simulink model "DT_GeneralFSM"  (R2025b)
settings: Solver=VariableStepAuto  StartTime=0.0  StopTime=1343.25  RelTol=1e-3
values from neighbouring files (symbols this model uses):
  feeddata = struct()    [DT_generatedata.m]    (also in DT_readdata.m)
  GSmode = input(['Choose the model type\n'                  '   [1] Kinetic + Genome-Scale Model\n'                  '   [2] Kinetic Only\n'                  'Response: '])    [DT_Run_GSA.m]    (also in DT_run.m; DT_run_OptimizeCOGs.m = 0; DT_run_ParaEst.m)
undefined symbols (not defined in the file or in its folder): V1, V2, V3, V4, V5, V6, V7
libraries: DT_Library x30
settings Model: DataDictionary=DT_types.sldd  SimulationMode=accelerator  PacingRate=0.100000  Creator=fenix  LastModifiedBy=Fenix
settings DebuggingCC: AlgebraicLoopMsg=error  UnitsInconsistencyMsg=none

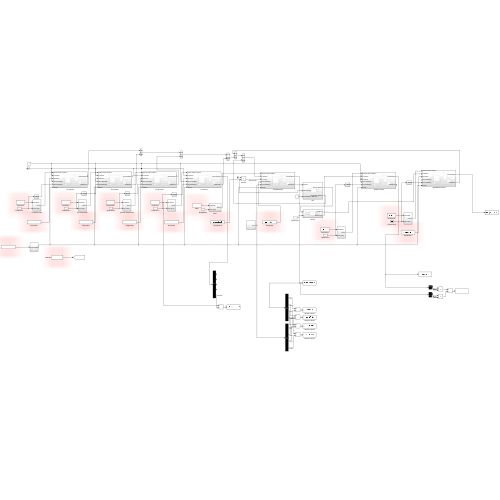
[thumbnail: Simulink's stored preview of the top-level diagram]
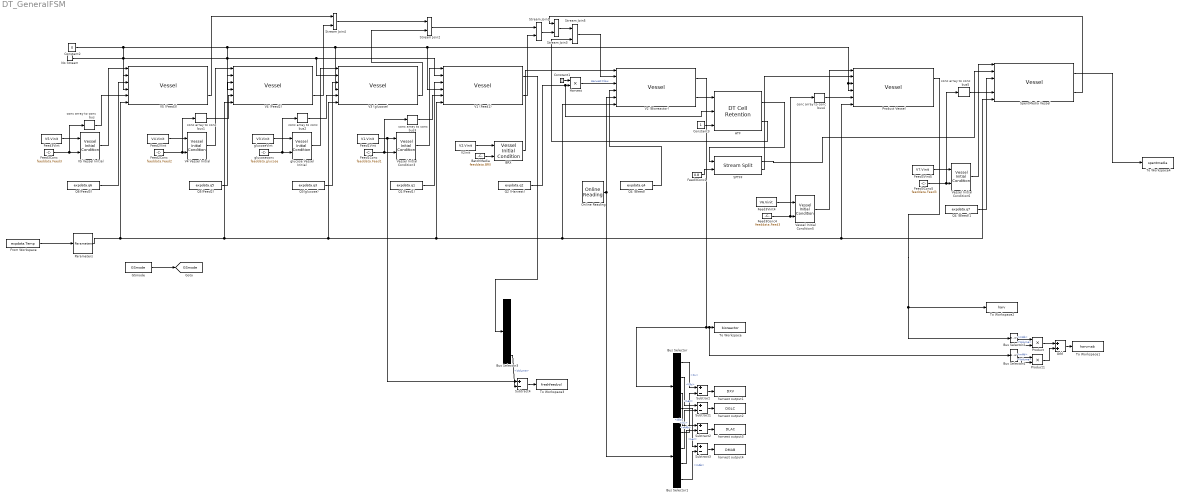
== system DT_GeneralFSM ==
  ATF : DT_Library/DT Cell Retention  SystemSampleTime=-1  VariantActivationTime=update diagram  EmptyChoice=off  PassThrough=off  PassThroughVariantControl=(default)  EmptyChoiceVariantControl=(default)  AllowFlexibleInterface=on  Latency=0  AutoFrameSizeCalculation=off
  Add : Sum
  BRX : DT_Library/Vessel Initial Condition  SystemSampleTime=-1  VariantActivationTime=update diagram  EmptyChoice=off  PassThrough=off  PassThroughVariantControl=(default)  EmptyChoiceVariantControl=(default)  AllowFlexibleInterface=on  Latency=0  AutoFrameSizeCalculation=off
  BatchMedia : Constant  Value=feeddata.BRX
  Bus Selector : BusSelector  OutputSignals=conc.Xv,conc.Glc,conc.Lac,conc.mAb
  Bus Selector1 : BusSelector  OutputSignals=Xv,Glc,Lac,mAb
  Bus Selector2 : BusSelector  OutputSignals=conc.Xv,conc.Glc,conc.Lac,conc.mAb,Volume
  Bus Selector3 : BusSelector  OutputSignals=conc.Xv,conc.Glc,conc.Lac,conc.mAb,Volume
  Bus Selector4 : BusSelector  OutputSignals=conc.Xv,conc.Glc,conc.Lac,conc.mAb,Volume
  Constant1 : Constant  Value=2
  Constant2 : Constant  Value=0
  Constant3 : Constant
  Feed1Conc : Constant  Value=feeddata.Feed1
  Feed1Vint : Constant  Value=V1.Vinit
  Feed2Conc : Constant  Value=feeddata.Feed2
  Feed2Vint : Constant  Value=V4.Vinit
  Feed3Conc : Constant  Value=feeddata.Feed3
  Feed3Conc1 : Constant  Value=0.8
  Feed3Conc4 : Constant  Value=feeddata.Feed3
  Feed3Conc5 : Constant  Value=feeddata.Feed3
  Feed3Vint : Constant  Value=V5.Vinit
  Feed3Vint4 : Constant  Value=V6.Vinit
  Feed3Vint5 : Constant  Value=V7.Vinit
  From Workspace : FromWorkspace  VariableName=expdata.Temp  Interpolate=off  OutputAfterFinalValue=Holding final value
  GSmode : Constant  Value=GSmode
  Harvest : Product
  No Stream : DT_Library/No Stream  SystemSampleTime=-1  VariantActivationTime=update diagram  EmptyChoice=off  PassThrough=off  PassThroughVariantControl=(default)  EmptyChoiceVariantControl=(default)  AllowFlexibleInterface=on  Latency=0  AutoFrameSizeCalculation=off
  Online Reading : DT_Library/Online Reading  SystemSampleTime=-1  VariantActivationTime=update diagram  EmptyChoice=off  PassThrough=off  PassThroughVariantControl=(default)  EmptyChoiceVariantControl=(default)  AllowFlexibleInterface=on  Latency=0  AutoFrameSizeCalculation=off
  Parameters : DT_Library/Parameters  SystemSampleTime=-1  VariantActivationTime=update diagram  EmptyChoice=off  PassThrough=off  PassThroughVariantControl=(default)  EmptyChoiceVariantControl=(default)  AllowFlexibleInterface=on  Latency=0  AutoFrameSizeCalculation=off
  Product : Product
  Product Vessel : DT_Library/Vessel  SystemSampleTime=-1  VariantActivationTime=update diagram  EmptyChoice=off  PassThrough=off  PassThroughVariantControl=(default)  EmptyChoiceVariantControl=(default)  AllowFlexibleInterface=on  Latency=0  AutoFrameSizeCalculation=off
  Product1 : Product
  Q1(Feed1) : FromWorkspace  VariableName=expdata.q1  Interpolate=off  OutputAfterFinalValue=Holding final value
  Q2 (Harvest) : FromWorkspace  VariableName=expdata.q2  Interpolate=off  OutputAfterFinalValue=Holding final value
  Q3(glucose) : FromWorkspace  VariableName=expdata.q3  Interpolate=off  OutputAfterFinalValue=Holding final value
  Q4 (Bleed) : FromWorkspace  VariableName=expdata.q4  Interpolate=off  OutputAfterFinalValue=Holding final value
  Q4 (Bleed)1 : FromWorkspace  VariableName=expdata.q7  Interpolate=off  OutputAfterFinalValue=Holding final value
  Q5(Feed2) : FromWorkspace  VariableName=expdata.q5  Interpolate=off  OutputAfterFinalValue=Holding final value
  Q6(Feed3) : FromWorkspace  VariableName=expdata.q6  Interpolate=off  OutputAfterFinalValue=Holding final value
  SPTFF : DT_Library/Stream Split  SystemSampleTime=-1  VariantActivationTime=update diagram  EmptyChoice=off  PassThrough=off  PassThroughVariantControl=(default)  EmptyChoiceVariantControl=(default)  AllowFlexibleInterface=on  Latency=0  AutoFrameSizeCalculation=off
  SpentMedia Vessel : DT_Library/Vessel  SystemSampleTime=-1  VariantActivationTime=update diagram  EmptyChoice=off  PassThrough=off  PassThroughVariantControl=(default)  EmptyChoiceVariantControl=(default)  AllowFlexibleInterface=on  Latency=0  AutoFrameSizeCalculation=off
  Stream Join{1..5} (5 alike) : DT_Library/Stream Join  SystemSampleTime=-1  VariantActivationTime=update diagram  EmptyChoice=off  PassThrough=off  PassThroughVariantControl=(default)  EmptyChoiceVariantControl=(default)  AllowFlexibleInterface=on  Latency=0  AutoFrameSizeCalculation=off
  Subtract{,1..4} (5 alike) : Sum  Inputs=+-
  To Workspace : ToWorkspace  VariableName=bioreactor  SaveFormat=Timeseries  SampleTime=-1
  To Workspace1 : ToWorkspace  VariableName=harvmab  SaveFormat=Timeseries  SampleTime=-1
  To Workspace2 : ToWorkspace  VariableName=harv  SaveFormat=Timeseries  SampleTime=-1
  To Workspace3 : ToWorkspace  VariableName=freshfeedvol  SaveFormat=Timeseries  SampleTime=-1
  To Workspace4 : ToWorkspace  VariableName=spentmedia  SaveFormat=Timeseries  SampleTime=-1
  V1 (Feed1) : DT_Library/Vessel  SystemSampleTime=-1  VariantActivationTime=update diagram  EmptyChoice=off  PassThrough=off  PassThroughVariantControl=(default)  EmptyChoiceVariantControl=(default)  AllowFlexibleInterface=on  Latency=0  AutoFrameSizeCalculation=off
  V2 (Bioreactor) : DT_Library/Vessel  SystemSampleTime=-1  VariantActivationTime=update diagram  EmptyChoice=off  PassThrough=off  PassThroughVariantControl=(default)  EmptyChoiceVariantControl=(default)  AllowFlexibleInterface=on  Latency=0  AutoFrameSizeCalculation=off
  V2init : Constant  Value=V2.Vinit
  V3 (glucose) : DT_Library/Vessel  SystemSampleTime=-1  VariantActivationTime=update diagram  EmptyChoice=off  PassThrough=off  PassThroughVariantControl=(default)  EmptyChoiceVariantControl=(default)  AllowFlexibleInterface=on  Latency=0  AutoFrameSizeCalculation=off
  V4 (Feed2) : DT_Library/Vessel  SystemSampleTime=-1  VariantActivationTime=update diagram  EmptyChoice=off  PassThrough=off  PassThroughVariantControl=(default)  EmptyChoiceVariantControl=(default)  AllowFlexibleInterface=on  Latency=0  AutoFrameSizeCalculation=off
  V4 Vessel Initial : DT_Library/Vessel Initial Condition  SystemSampleTime=-1  VariantActivationTime=update diagram  EmptyChoice=off  PassThrough=off  PassThroughVariantControl=(default)  EmptyChoiceVariantControl=(default)  AllowFlexibleInterface=on  Latency=0  AutoFrameSizeCalculation=off
  V5 (Feed3) : DT_Library/Vessel  SystemSampleTime=-1  VariantActivationTime=update diagram  EmptyChoice=off  PassThrough=off  PassThroughVariantControl=(default)  EmptyChoiceVariantControl=(default)  AllowFlexibleInterface=on  Latency=0  AutoFrameSizeCalculation=off
  "V5 Vessel Initial " : DT_Library/Vessel Initial Condition  SystemSampleTime=-1  VariantActivationTime=update diagram  EmptyChoice=off  PassThrough=off  PassThroughVariantControl=(default)  EmptyChoiceVariantControl=(default)  AllowFlexibleInterface=on  Latency=0  AutoFrameSizeCalculation=off
  Vessel Initial Condition3 : DT_Library/Vessel Initial Condition  SystemSampleTime=-1  VariantActivationTime=update diagram  EmptyChoice=off  PassThrough=off  PassThroughVariantControl=(default)  EmptyChoiceVariantControl=(default)  AllowFlexibleInterface=on  Latency=0  AutoFrameSizeCalculation=off
  Vessel Initial Condition5 : DT_Library/Vessel Initial Condition  SystemSampleTime=-1  VariantActivationTime=update diagram  EmptyChoice=off  PassThrough=off  PassThroughVariantControl=(default)  EmptyChoiceVariantControl=(default)  AllowFlexibleInterface=on  Latency=0  AutoFrameSizeCalculation=off
  Vessel Initial Condition6 : DT_Library/Vessel Initial Condition  SystemSampleTime=-1  VariantActivationTime=update diagram  EmptyChoice=off  PassThrough=off  PassThroughVariantControl=(default)  EmptyChoiceVariantControl=(default)  AllowFlexibleInterface=on  Latency=0  AutoFrameSizeCalculation=off
  conc array to conc bus{,1..5} (6 alike) : DT_Library/conc array to conc bus  SystemSampleTime=-1  VariantActivationTime=update diagram  EmptyChoice=off  PassThrough=off  PassThroughVariantControl=(default)  EmptyChoiceVariantControl=(default)  AllowFlexibleInterface=on  Latency=0  AutoFrameSizeCalculation=off
  glucose Vessel Initial : DT_Library/Vessel Initial Condition  SystemSampleTime=-1  VariantActivationTime=update diagram  EmptyChoice=off  PassThrough=off  PassThroughVariantControl=(default)  EmptyChoiceVariantControl=(default)  AllowFlexibleInterface=on  Latency=0  AutoFrameSizeCalculation=off
  glucoseVint : Constant  Value=V3.Vinit
  glucoseconc : Constant  Value=feeddata.glucose
  harvest output1 : ToWorkspace  VariableName=DXV  SaveFormat=Timeseries  SampleTime=-1
  harvest output2 : ToWorkspace  VariableName=DGLC  SaveFormat=Timeseries  SampleTime=-1
  harvest output3 : ToWorkspace  VariableName=DLAC  SaveFormat=Timeseries  SampleTime=-1
  harvest output4 : ToWorkspace  VariableName=DMAB  SaveFormat=Timeseries  SampleTime=-1
  tag scope: GSmode=global
  wires:
  BatchMedia/1 -> BRX/2
  V2init/1 -> BRX/1
  BRX/1 -> V2 (Bioreactor)/1
  Online Reading/1 -> Bus Selector1/1, V2 (Bioreactor)/5
  Q2 (Harvest)/1 -> ATF/2, Harvest/2
  Q4 (Bleed)/1 -> V2 (Bioreactor)/4
  From Workspace/1 -> Parameters/1
  Parameters/1 -> V5 (Feed3)/6, V1 (Feed1)/6, Product Vessel/6, SpentMedia Vessel/6, V2 (Bioreactor)/6, V3 (glucose)/6, V4 (Feed2)/6
  V1 (Feed1)/2 -> Stream Join1/2
  V3 (glucose)/2 -> Stream Join2/2
  Stream Join2/1 -> Stream Join1/1
  V2 (Bioreactor)/2 -> ATF/1
  Constant1/1 -> Harvest/1
  Harvest/1 -> V2 (Bioreactor)/3  "Harvest Flow"
  Constant3/1 -> ATF/3
  ATF/1 -> SPTFF/1
  Q4 (Bleed)1/1 -> SpentMedia Vessel/3
  SpentMedia Vessel/2 -> Stream Join3/1
  SPTFF/1 -> SpentMedia Vessel/2
  Stream Join4/1 -> Stream Join2/1
  V4 (Feed2)/2 -> Stream Join4/2
  V5 (Feed3)/2 -> Stream Join4/1
  Q6(Feed3)/1 -> V5 (Feed3)/3
  Q5(Feed2)/1 -> V4 (Feed2)/3
  Q3(glucose)/1 -> V3 (glucose)/3
  Q1(Feed1)/1 -> V1 (Feed1)/3
  Feed3Vint/1 -> "V5 Vessel Initial "/1
  Feed3Conc/1 -> conc array to conc bus/1, "V5 Vessel Initial "/2
  "V5 Vessel Initial "/1 -> V5 (Feed3)/1
  Feed2Conc/1 -> conc array to conc bus1/1, V4 Vessel Initial/2
  V4 Vessel Initial/1 -> V4 (Feed2)/1
  glucoseconc/1 -> conc array to conc bus2/1, glucose Vessel Initial/2
  glucose Vessel Initial/1 -> V3 (glucose)/1
  Feed1Conc/1 -> conc array to conc bus3/1, Vessel Initial Condition3/2
  Vessel Initial Condition3/1 -> V1 (Feed1)/1
  Feed3Conc4/1 -> conc array to conc bus4/1, Vessel Initial Condition5/2
  Vessel Initial Condition5/1 -> Product Vessel/1
  Feed3Vint4/1 -> Vessel Initial Condition5/1
  Feed1Vint/1 -> Subtract4/1, Vessel Initial Condition3/1
  glucoseVint/1 -> glucose Vessel Initial/1
  Feed2Vint/1 -> V4 Vessel Initial/1
  Feed3Vint5/1 -> Vessel Initial Condition6/1
  Feed3Conc5/1 -> conc array to conc bus5/1, Vessel Initial Condition6/2
  Vessel Initial Condition6/1 -> SpentMedia Vessel/1
  Stream Join3/1 -> Stream Join5/1
  ATF/2 -> Stream Join5/2
  Stream Join5/1 -> V2 (Bioreactor)/2
  No Stream/1 -> V5 (Feed3)/2, V1 (Feed1)/2, V3 (glucose)/2, V4 (Feed2)/2
  conc array to conc bus/1 -> V5 (Feed3)/5
  conc array to conc bus1/1 -> V4 (Feed2)/5
  conc array to conc bus2/1 -> V3 (glucose)/5
  conc array to conc bus3/1 -> V1 (Feed1)/5
  conc array to conc bus4/1 -> Product Vessel/5
  conc array to conc bus5/1 -> SpentMedia Vessel/5
  Constant2/1 -> V4 (Feed2)/4, V3 (glucose)/4, V1 (Feed1)/4, Product Vessel/4, Product Vessel/3, V5 (Feed3)/4
  Subtract/1 -> harvest output1/1
  Subtract1/1 -> harvest output2/1
  Subtract2/1 -> harvest output3/1
  Subtract3/1 -> harvest output4/1
  Bus Selector/1 -> Subtract/1  "<Xv>"
  Bus Selector1/1 -> Subtract/2  "<Xv>"
  Bus Selector/2 -> Subtract1/1  "<Glc>"
  Bus Selector1/2 -> Subtract1/2  "<Glc>"
  Bus Selector/3 -> Subtract2/1  "<Lac>"
  Bus Selector1/3 -> Subtract2/2  "<Lac>"
  Bus Selector/4 -> Subtract3/1  "<mAb>"
  Bus Selector1/4 -> Subtract3/2  "<mAb>"
  Stream Join1/1 -> Stream Join3/2
  Product Vessel/1 -> To Workspace2/1, Bus Selector2/1
  Bus Selector2/4 -> Product/1  "<mAb>"
  Bus Selector2/5 -> Product/2  "<Volume>"
  Product/1 -> Add/1
  SPTFF/2 -> Product Vessel/2
  V1 (Feed1)/1 -> Bus Selector3/1
  Bus Selector3/5 -> Subtract4/2  "<Volume>"
  Subtract4/1 -> To Workspace3/1
  GSmode/1 -> [GSmode]
  V2 (Bioreactor)/1 -> To Workspace/1, Bus Selector4/1, Bus Selector/1
  Bus Selector4/5 -> Product1/2  "<Volume>"
  Bus Selector4/4 -> Product1/1  "<mAb>"
  Product1/1 -> Add/2
  Add/1 -> To Workspace1/1
  SpentMedia Vessel/1 -> To Workspace4/1
  Feed3Conc1/1 -> SPTFF/2
